simulink model "blending_tank_auto"  (R2020b)
settings: Solver=FixedStepAuto  StartTime=0.0  StopTime=Inf  RelTol=1e-3
PostLoadFcn:
  | slplc.api.loadDataTypes;
InitFcn:
  | T1_InitialValue = FB_TON.InitialValue;
  | T1_InitialValue.PRE = 20000;
  | 
  | C1_InitialValue = FB_CTU.InitialValue;
  | C1_InitialValue.PRE = 3;
StopFcn:
  | clear T1_InitialValue C1_InitialValue;
undefined symbols (not defined in the file): BOOL, DINT, OTL, REAL, slplc
libraries: simulink x3, sldrtlib x1
(part 11 of 15)

== system blending_tank_auto/PLC Controller/__Logic/Task/Program/__Logic/OTU7/Instruction_Enable/Rung-condition-in is true ==
  Enable : EnablePort
  Constant : Constant  Value=0  OutDataTypeStr=BOOL
  __CoreVarWrite : Subsystem  Tag=CoreVarWriteBlock  DisableCoverage=on  TreatAsAtomicUnit=on  mask{PLCBlockType=CoreVarWrite}
      mask init:
      | slplc.callbacks.initCoreVariable(gcb, 'write');
      mask Help: web([docroot '/plccoder/ref/__corevarwrite' '.html']);
      mask DialogControl PLCBlockTitle Prompt: Core Variable Write
  wires:
  Constant/1 -> __CoreVarWrite/1(u)

== system blending_tank_auto/PLC Controller/__Logic/Task/Program/__Logic/OTU7/RungInOverride/ForceRungInFalseRead ==
  __CoreLabelRead : Subsystem  Tag=CoreVarReadBlock  DisableCoverage=on  TreatAsAtomicUnit=on  mask{PLCBlockType=CoreLabelRead}
      mask init:
      | slplc.callbacks.initRoutineLabelRead(gcb);
      mask Help: web([docroot '/plccoder/ref/__corelabelread' '.html']);
      mask DialogControl PLCBlockTitle Prompt: Core Label Read
  Out1 : Outport  VectorParamsAs1DForOutWhenUnconnected=off
  wires:
  __CoreLabelRead/1(Out1) -> Out1/1

== system blending_tank_auto/PLC Controller/__Logic/Task/Program/__Logic/OTU8/BlockEnableRead/__CoreLabelRead ==
  DataRead : DataStoreRead  DataStoreName=x_PLCLabel__s4_3653__Block_Enable
  Out1 : Outport  VectorParamsAs1DForOutWhenUnconnected=off
  wires:
  DataRead/1 -> Out1/1

== system blending_tank_auto/PLC Controller/__Logic/Task/Program/__Logic/OTU8/Instruction_Enable/Rung-condition-in is true ==
  Enable : EnablePort
  Constant : Constant  Value=0  OutDataTypeStr=BOOL
  __CoreVarWrite : Subsystem  Tag=CoreVarWriteBlock  DisableCoverage=on  TreatAsAtomicUnit=on  mask{PLCBlockType=CoreVarWrite}
      mask init:
      | slplc.callbacks.initCoreVariable(gcb, 'write');
      mask Help: web([docroot '/plccoder/ref/__corevarwrite' '.html']);
      mask DialogControl PLCBlockTitle Prompt: Core Variable Write
  wires:
  Constant/1 -> __CoreVarWrite/1(u)

== system blending_tank_auto/PLC Controller/__Logic/Task/Program/__Logic/OTU8/RungInOverride/ForceRungInFalseRead ==
  __CoreLabelRead : Subsystem  Tag=CoreVarReadBlock  DisableCoverage=on  TreatAsAtomicUnit=on  mask{PLCBlockType=CoreLabelRead}
      mask init:
      | slplc.callbacks.initRoutineLabelRead(gcb);
      mask Help: web([docroot '/plccoder/ref/__corelabelread' '.html']);
      mask DialogControl PLCBlockTitle Prompt: Core Label Read
  Out1 : Outport  VectorParamsAs1DForOutWhenUnconnected=off
  wires:
  __CoreLabelRead/1(Out1) -> Out1/1

== system blending_tank_auto/PLC Controller/__Logic/Task/Program/__Logic/OTU9/BlockEnableRead/__CoreLabelRead ==
  DataRead : DataStoreRead  DataStoreName=x_PLCLabel__s4_3653__Block_Enable
  Out1 : Outport  VectorParamsAs1DForOutWhenUnconnected=off
  wires:
  DataRead/1 -> Out1/1

== system blending_tank_auto/PLC Controller/__Logic/Task/Program/__Logic/OTU9/Instruction_Enable/Rung-condition-in is true ==
  Enable : EnablePort
  Constant : Constant  Value=0  OutDataTypeStr=BOOL
  __CoreVarWrite : Subsystem  Tag=CoreVarWriteBlock  DisableCoverage=on  TreatAsAtomicUnit=on  mask{PLCBlockType=CoreVarWrite}
      mask init:
      | slplc.callbacks.initCoreVariable(gcb, 'write');
      mask Help: web([docroot '/plccoder/ref/__corevarwrite' '.html']);
      mask DialogControl PLCBlockTitle Prompt: Core Variable Write
  wires:
  Constant/1 -> __CoreVarWrite/1(u)

== system blending_tank_auto/PLC Controller/__Logic/Task/Program/__Logic/OTU9/RungInOverride/ForceRungInFalseRead ==
  __CoreLabelRead : Subsystem  Tag=CoreVarReadBlock  DisableCoverage=on  TreatAsAtomicUnit=on  mask{PLCBlockType=CoreLabelRead}
      mask init:
      | slplc.callbacks.initRoutineLabelRead(gcb);
      mask Help: web([docroot '/plccoder/ref/__corelabelread' '.html']);
      mask DialogControl PLCBlockTitle Prompt: Core Label Read
  Out1 : Outport  VectorParamsAs1DForOutWhenUnconnected=off
  wires:
  __CoreLabelRead/1(Out1) -> Out1/1

== system blending_tank_auto/PLC Controller/__Logic/Task/Program/__Logic/RES/BlockEnableRead/__CoreLabelRead ==
  DataRead : DataStoreRead  DataStoreName=x_PLCLabel__s4_3653__Block_Enable
  Out1 : Outport  VectorParamsAs1DForOutWhenUnconnected=off
  wires:
  DataRead/1 -> Out1/1

== system blending_tank_auto/PLC Controller/__Logic/Task/Program/__Logic/RES/Instruction_Enable/Rung-condition-in is true ==
  Enable : EnablePort
  __CoreVarRead : Subsystem  Tag=CoreVarReadBlock  DisableCoverage=on  TreatAsAtomicUnit=on  mask{PLCBlockType=CoreVarRead}
      mask init:
      | slplc.callbacks.initCoreVariable(gcb, 'read');
      mask Help: web([docroot '/plccoder/ref/__corevarread' '.html']);
      mask DialogControl PLCBlockTitle Prompt: Core Variable Read
  __CoreVarWrite : Subsystem  Tag=CoreVarWriteBlock  DisableCoverage=on  TreatAsAtomicUnit=on  mask{PLCBlockType=CoreVarWrite}
      mask init:
      | slplc.callbacks.initCoreVariable(gcb, 'write');
      mask Help: web([docroot '/plccoder/ref/__corevarwrite' '.html']);
      mask DialogControl PLCBlockTitle Prompt: Core Variable Write
  reset_function : MATLAB Function  DisableCoverage=on  TreatAsAtomicUnit=on
  wires:
  __CoreVarRead/1(y) -> reset_function/1("y ")
  reset_function/1(y) -> __CoreVarWrite/1(u)

== system blending_tank_auto/PLC Controller/__Logic/Task/Program/__Logic/RES/RungInOverride/ForceRungInFalseRead ==
  __CoreLabelRead : Subsystem  Tag=CoreVarReadBlock  DisableCoverage=on  TreatAsAtomicUnit=on  mask{PLCBlockType=CoreLabelRead}
      mask init:
      | slplc.callbacks.initRoutineLabelRead(gcb);
      mask Help: web([docroot '/plccoder/ref/__corelabelread' '.html']);
      mask DialogControl PLCBlockTitle Prompt: Core Label Read
  Out1 : Outport  VectorParamsAs1DForOutWhenUnconnected=off
  wires:
  __CoreLabelRead/1(Out1) -> Out1/1

== system blending_tank_auto/PLC Controller/__Logic/Task/Program/__Logic/RES1/BlockEnableRead/__CoreLabelRead ==
  DataRead : DataStoreRead  DataStoreName=x_PLCLabel__s4_3653__Block_Enable
  Out1 : Outport  VectorParamsAs1DForOutWhenUnconnected=off
  wires:
  DataRead/1 -> Out1/1

== system blending_tank_auto/PLC Controller/__Logic/Task/Program/__Logic/RES1/Instruction_Enable/Rung-condition-in is true ==
  Enable : EnablePort
  __CoreVarRead : Subsystem  Tag=CoreVarReadBlock  DisableCoverage=on  TreatAsAtomicUnit=on  mask{PLCBlockType=CoreVarRead}
      mask init:
      | slplc.callbacks.initCoreVariable(gcb, 'read');
      mask Help: web([docroot '/plccoder/ref/__corevarread' '.html']);
      mask DialogControl PLCBlockTitle Prompt: Core Variable Read
  __CoreVarWrite : Subsystem  Tag=CoreVarWriteBlock  DisableCoverage=on  TreatAsAtomicUnit=on  mask{PLCBlockType=CoreVarWrite}
      mask init:
      | slplc.callbacks.initCoreVariable(gcb, 'write');
      mask Help: web([docroot '/plccoder/ref/__corevarwrite' '.html']);
      mask DialogControl PLCBlockTitle Prompt: Core Variable Write
  reset_function : MATLAB Function  DisableCoverage=on  TreatAsAtomicUnit=on
  wires:
  __CoreVarRead/1(y) -> reset_function/1("y ")
  reset_function/1(y) -> __CoreVarWrite/1(u)

== system blending_tank_auto/PLC Controller/__Logic/Task/Program/__Logic/RES1/RungInOverride/ForceRungInFalseRead ==
  __CoreLabelRead : Subsystem  Tag=CoreVarReadBlock  DisableCoverage=on  TreatAsAtomicUnit=on  mask{PLCBlockType=CoreLabelRead}
      mask init:
      | slplc.callbacks.initRoutineLabelRead(gcb);
      mask Help: web([docroot '/plccoder/ref/__corelabelread' '.html']);
      mask DialogControl PLCBlockTitle Prompt: Core Label Read
  Out1 : Outport  VectorParamsAs1DForOutWhenUnconnected=off
  wires:
  __CoreLabelRead/1(Out1) -> Out1/1

== system blending_tank_auto/PLC Controller/__Logic/Task/Program/__Logic/TON/BlockEnableRead/__CoreLabelRead ==
  DataRead : DataStoreRead  DataStoreName=x_PLCLabel__s4_3653__Block_Enable
  Out1 : Outport  VectorParamsAs1DForOutWhenUnconnected=off
  wires:
  DataRead/1 -> Out1/1

== system blending_tank_auto/PLC Controller/__Logic/Task/Program/__Logic/TON/Instruction_Enable/Initialize Function ==
  Constant : Constant  Value=0  OutDataTypeStr=BOOL
  Constant1 : Constant  Value=0  OutDataTypeStr=DINT
  Event Listener : EventListener  DisableCoverage=on  EventName=reset
  VarWrite : Subsystem  DisableCoverage=on  TreatAsAtomicUnit=on  mask{PLCOperandTag=ACC, PLCOperandExpression=xxx_PLC_VAR_T1.ACC, PLCBlockType=VarWrite, PLCPOUType=VarWrite}
      mask prompts: PLCOperandTag "Operand Tag:"
      mask init:
      | slplc.callbacks.initInstruction(gcb);
      mask Help: web([docroot '/plccoder/ref/varwrite' '.html']);
      mask DialogControl PLCBlockTitle Prompt: Variable Write
      mask Display: disp(get_param(gcb, 'PLCOperandTag'));
  VarWrite1 : Subsystem  DisableCoverage=on  TreatAsAtomicUnit=on  mask{PLCOperandTag=EN, PLCOperandExpression=xxx_PLC_VAR_T1.EN, PLCBlockType=VarWrite, PLCPOUType=VarWrite}
      mask prompts: PLCOperandTag "Operand Tag:"
      mask init:
      | slplc.callbacks.initInstruction(gcb);
      mask Help: web([docroot '/plccoder/ref/varwrite' '.html']);
      mask DialogControl PLCBlockTitle Prompt: Variable Write
      mask Display: disp(get_param(gcb, 'PLCOperandTag'));
  VarWrite2 : Subsystem  DisableCoverage=on  TreatAsAtomicUnit=on  mask{PLCOperandTag=TT, PLCOperandExpression=xxx_PLC_VAR_T1.TT, PLCBlockType=VarWrite, PLCPOUType=VarWrite}
      mask prompts: PLCOperandTag "Operand Tag:"
      mask init:
      | slplc.callbacks.initInstruction(gcb);
      mask Help: web([docroot '/plccoder/ref/varwrite' '.html']);
      mask DialogControl PLCBlockTitle Prompt: Variable Write
      mask Display: disp(get_param(gcb, 'PLCOperandTag'));
  VarWrite3 : Subsystem  DisableCoverage=on  TreatAsAtomicUnit=on  mask{PLCOperandTag=DN, PLCOperandExpression=xxx_PLC_VAR_T1.DN, PLCBlockType=VarWrite, PLCPOUType=VarWrite}
      mask prompts: PLCOperandTag "Operand Tag:"
      mask init:
      | slplc.callbacks.initInstruction(gcb);
      mask Help: web([docroot '/plccoder/ref/varwrite' '.html']);
      mask DialogControl PLCBlockTitle Prompt: Variable Write
      mask Display: disp(get_param(gcb, 'PLCOperandTag'));
  wires:
  Constant/1 -> VarWrite1/1(In1), VarWrite2/1(In1), VarWrite3/1(In1)
  Constant1/1 -> VarWrite/1(In1)

== system blending_tank_auto/PLC Controller/__Logic/Task/Program/__Logic/TON/Instruction_Enable/__CoreVarRead ==
  DataRead : DataStoreRead  DataStoreName=xxx_PLC_VAR_T1
  y : Outport  VectorParamsAs1DForOutWhenUnconnected=off
  wires:
  DataRead/1 -> y/1

== system blending_tank_auto/PLC Controller/__Logic/Task/Program/__Logic/TON/Instruction_Enable/__CoreVarWrite ==
  u : Inport
  DataWrite : DataStoreWrite  DataStoreName=xxx_PLC_VAR_T1
  wires:
  u/1 -> DataWrite/1

== system blending_tank_auto/PLC Controller/__Logic/Task/Program/__Logic/TON/RungInOverride/ForceRungInFalseRead ==
  __CoreLabelRead : Subsystem  Tag=CoreVarReadBlock  DisableCoverage=on  TreatAsAtomicUnit=on  mask{PLCBlockType=CoreLabelRead}
      mask init:
      | slplc.callbacks.initRoutineLabelRead(gcb);
      mask Help: web([docroot '/plccoder/ref/__corelabelread' '.html']);
      mask DialogControl PLCBlockTitle Prompt: Core Label Read
  Out1 : Outport  VectorParamsAs1DForOutWhenUnconnected=off
  wires:
  __CoreLabelRead/1(Out1) -> Out1/1

== system blending_tank_auto/PLC Controller/__Logic/Task/Program/__Logic/XIC/BlockEnableRead/__CoreLabelRead ==
  DataRead : DataStoreRead  DataStoreName=x_PLCLabel__s4_3653__Block_Enable
  Out1 : Outport  VectorParamsAs1DForOutWhenUnconnected=off
  wires:
  DataRead/1 -> Out1/1

== system blending_tank_auto/PLC Controller/__Logic/Task/Program/__Logic/XIC/Instruction_Enable/__CoreVarRead ==
  DataRead : DataStoreRead  DataStoreName=xxx_PLC_VAR_Initialise
  y : Outport  VectorParamsAs1DForOutWhenUnconnected=off
  wires:
  DataRead/1 -> y/1

== system blending_tank_auto/PLC Controller/__Logic/Task/Program/__Logic/XIC/RungInOverride/ForceRungInFalseRead ==
  __CoreLabelRead : Subsystem  Tag=CoreVarReadBlock  DisableCoverage=on  TreatAsAtomicUnit=on  mask{PLCBlockType=CoreLabelRead}
      mask init:
      | slplc.callbacks.initRoutineLabelRead(gcb);
      mask Help: web([docroot '/plccoder/ref/__corelabelread' '.html']);
      mask DialogControl PLCBlockTitle Prompt: Core Label Read
  Out1 : Outport  VectorParamsAs1DForOutWhenUnconnected=off
  wires:
  __CoreLabelRead/1(Out1) -> Out1/1

== system blending_tank_auto/PLC Controller/__Logic/Task/Program/__Logic/XIC1/BlockEnableRead/__CoreLabelRead ==
  DataRead : DataStoreRead  DataStoreName=x_PLCLabel__s4_3653__Block_Enable
  Out1 : Outport  VectorParamsAs1DForOutWhenUnconnected=off
  wires:
  DataRead/1 -> Out1/1

== system blending_tank_auto/PLC Controller/__Logic/Task/Program/__Logic/XIC1/Instruction_Enable/__CoreVarRead ==
  DataRead : DataStoreRead  DataStoreName=xxx_PLC_VAR_M0
  y : Outport  VectorParamsAs1DForOutWhenUnconnected=off
  wires:
  DataRead/1 -> y/1

== system blending_tank_auto/PLC Controller/__Logic/Task/Program/__Logic/XIC1/RungInOverride/ForceRungInFalseRead ==
  __CoreLabelRead : Subsystem  Tag=CoreVarReadBlock  DisableCoverage=on  TreatAsAtomicUnit=on  mask{PLCBlockType=CoreLabelRead}
      mask init:
      | slplc.callbacks.initRoutineLabelRead(gcb);
      mask Help: web([docroot '/plccoder/ref/__corelabelread' '.html']);
      mask DialogControl PLCBlockTitle Prompt: Core Label Read
  Out1 : Outport  VectorParamsAs1DForOutWhenUnconnected=off
  wires:
  __CoreLabelRead/1(Out1) -> Out1/1

== system blending_tank_auto/PLC Controller/__Logic/Task/Program/__Logic/XIC10/BlockEnableRead/__CoreLabelRead ==
  DataRead : DataStoreRead  DataStoreName=x_PLCLabel__s4_3653__Block_Enable
  Out1 : Outport  VectorParamsAs1DForOutWhenUnconnected=off
  wires:
  DataRead/1 -> Out1/1

== system blending_tank_auto/PLC Controller/__Logic/Task/Program/__Logic/XIC10/Instruction_Enable/__CoreVarRead ==
  DataRead : DataStoreRead  DataStoreName=xxx_PLC_VAR_M6
  y : Outport  VectorParamsAs1DForOutWhenUnconnected=off
  wires:
  DataRead/1 -> y/1

== system blending_tank_auto/PLC Controller/__Logic/Task/Program/__Logic/XIC10/RungInOverride/ForceRungInFalseRead ==
  __CoreLabelRead : Subsystem  Tag=CoreVarReadBlock  DisableCoverage=on  TreatAsAtomicUnit=on  mask{PLCBlockType=CoreLabelRead}
      mask init:
      | slplc.callbacks.initRoutineLabelRead(gcb);
      mask Help: web([docroot '/plccoder/ref/__corelabelread' '.html']);
      mask DialogControl PLCBlockTitle Prompt: Core Label Read
  Out1 : Outport  VectorParamsAs1DForOutWhenUnconnected=off
  wires:
  __CoreLabelRead/1(Out1) -> Out1/1

== system blending_tank_auto/PLC Controller/__Logic/Task/Program/__Logic/XIC11/BlockEnableRead/__CoreLabelRead ==
  DataRead : DataStoreRead  DataStoreName=x_PLCLabel__s4_3653__Block_Enable
  Out1 : Outport  VectorParamsAs1DForOutWhenUnconnected=off
  wires:
  DataRead/1 -> Out1/1

== system blending_tank_auto/PLC Controller/__Logic/Task/Program/__Logic/XIC11/Instruction_Enable/__CoreVarRead ==
  DataRead : DataStoreRead  DataStoreName=xxx_PLC_VAR_M7
  y : Outport  VectorParamsAs1DForOutWhenUnconnected=off
  wires:
  DataRead/1 -> y/1

== system blending_tank_auto/PLC Controller/__Logic/Task/Program/__Logic/XIC11/RungInOverride/ForceRungInFalseRead ==
  __CoreLabelRead : Subsystem  Tag=CoreVarReadBlock  DisableCoverage=on  TreatAsAtomicUnit=on  mask{PLCBlockType=CoreLabelRead}
      mask init:
      | slplc.callbacks.initRoutineLabelRead(gcb);
      mask Help: web([docroot '/plccoder/ref/__corelabelread' '.html']);
      mask DialogControl PLCBlockTitle Prompt: Core Label Read
  Out1 : Outport  VectorParamsAs1DForOutWhenUnconnected=off
  wires:
  __CoreLabelRead/1(Out1) -> Out1/1

== system blending_tank_auto/PLC Controller/__Logic/Task/Program/__Logic/XIC12/BlockEnableRead/__CoreLabelRead ==
  DataRead : DataStoreRead  DataStoreName=x_PLCLabel__s4_3653__Block_Enable
  Out1 : Outport  VectorParamsAs1DForOutWhenUnconnected=off
  wires:
  DataRead/1 -> Out1/1

== system blending_tank_auto/PLC Controller/__Logic/Task/Program/__Logic/XIC12/Instruction_Enable/__CoreVarRead ==
  DataRead : DataStoreRead  DataStoreName=xxx_PLC_VAR_M5
  y : Outport  VectorParamsAs1DForOutWhenUnconnected=off
  wires:
  DataRead/1 -> y/1

== system blending_tank_auto/PLC Controller/__Logic/Task/Program/__Logic/XIC12/RungInOverride/ForceRungInFalseRead ==
  __CoreLabelRead : Subsystem  Tag=CoreVarReadBlock  DisableCoverage=on  TreatAsAtomicUnit=on  mask{PLCBlockType=CoreLabelRead}
      mask init:
      | slplc.callbacks.initRoutineLabelRead(gcb);
      mask Help: web([docroot '/plccoder/ref/__corelabelread' '.html']);
      mask DialogControl PLCBlockTitle Prompt: Core Label Read
  Out1 : Outport  VectorParamsAs1DForOutWhenUnconnected=off
  wires:
  __CoreLabelRead/1(Out1) -> Out1/1

== system blending_tank_auto/PLC Controller/__Logic/Task/Program/__Logic/XIC13/BlockEnableRead/__CoreLabelRead ==
  DataRead : DataStoreRead  DataStoreName=x_PLCLabel__s4_3653__Block_Enable
  Out1 : Outport  VectorParamsAs1DForOutWhenUnconnected=off
  wires:
  DataRead/1 -> Out1/1

== system blending_tank_auto/PLC Controller/__Logic/Task/Program/__Logic/XIC13/Instruction_Enable/__CoreVarRead ==
  DataRead : DataStoreRead  DataStoreName=xxx_PLC_VAR_M2
  y : Outport  VectorParamsAs1DForOutWhenUnconnected=off
  wires:
  DataRead/1 -> y/1

== system blending_tank_auto/PLC Controller/__Logic/Task/Program/__Logic/XIC13/RungInOverride/ForceRungInFalseRead ==
  __CoreLabelRead : Subsystem  Tag=CoreVarReadBlock  DisableCoverage=on  TreatAsAtomicUnit=on  mask{PLCBlockType=CoreLabelRead}
      mask init:
      | slplc.callbacks.initRoutineLabelRead(gcb);
      mask Help: web([docroot '/plccoder/ref/__corelabelread' '.html']);
      mask DialogControl PLCBlockTitle Prompt: Core Label Read
  Out1 : Outport  VectorParamsAs1DForOutWhenUnconnected=off
  wires:
  __CoreLabelRead/1(Out1) -> Out1/1

== system blending_tank_auto/PLC Controller/__Logic/Task/Program/__Logic/XIC14/BlockEnableRead/__CoreLabelRead ==
  DataRead : DataStoreRead  DataStoreName=x_PLCLabel__s4_3653__Block_Enable
  Out1 : Outport  VectorParamsAs1DForOutWhenUnconnected=off
  wires:
  DataRead/1 -> Out1/1

== system blending_tank_auto/PLC Controller/__Logic/Task/Program/__Logic/XIC14/Instruction_Enable/__CoreVarRead ==
  DataRead : DataStoreRead  DataStoreName=xxx_PLC_VAR_M3
  y : Outport  VectorParamsAs1DForOutWhenUnconnected=off
  wires:
  DataRead/1 -> y/1

== system blending_tank_auto/PLC Controller/__Logic/Task/Program/__Logic/XIC14/RungInOverride/ForceRungInFalseRead ==
  __CoreLabelRead : Subsystem  Tag=CoreVarReadBlock  DisableCoverage=on  TreatAsAtomicUnit=on  mask{PLCBlockType=CoreLabelRead}
      mask init:
      | slplc.callbacks.initRoutineLabelRead(gcb);
      mask Help: web([docroot '/plccoder/ref/__corelabelread' '.html']);
      mask DialogControl PLCBlockTitle Prompt: Core Label Read
  Out1 : Outport  VectorParamsAs1DForOutWhenUnconnected=off
  wires:
  __CoreLabelRead/1(Out1) -> Out1/1

== system blending_tank_auto/PLC Controller/__Logic/Task/Program/__Logic/XIC15/BlockEnableRead/__CoreLabelRead ==
  DataRead : DataStoreRead  DataStoreName=x_PLCLabel__s4_3653__Block_Enable
  Out1 : Outport  VectorParamsAs1DForOutWhenUnconnected=off
  wires:
  DataRead/1 -> Out1/1

== system blending_tank_auto/PLC Controller/__Logic/Task/Program/__Logic/XIC15/Instruction_Enable/__CoreVarRead ==
  DataRead : DataStoreRead  DataStoreName=xxx_PLC_VAR_M4
  y : Outport  VectorParamsAs1DForOutWhenUnconnected=off
  wires:
  DataRead/1 -> y/1

== system blending_tank_auto/PLC Controller/__Logic/Task/Program/__Logic/XIC15/RungInOverride/ForceRungInFalseRead ==
  __CoreLabelRead : Subsystem  Tag=CoreVarReadBlock  DisableCoverage=on  TreatAsAtomicUnit=on  mask{PLCBlockType=CoreLabelRead}
      mask init:
      | slplc.callbacks.initRoutineLabelRead(gcb);
      mask Help: web([docroot '/plccoder/ref/__corelabelread' '.html']);
      mask DialogControl PLCBlockTitle Prompt: Core Label Read
  Out1 : Outport  VectorParamsAs1DForOutWhenUnconnected=off
  wires:
  __CoreLabelRead/1(Out1) -> Out1/1

== system blending_tank_auto/PLC Controller/__Logic/Task/Program/__Logic/XIC16/BlockEnableRead/__CoreLabelRead ==
  DataRead : DataStoreRead  DataStoreName=x_PLCLabel__s4_3653__Block_Enable
  Out1 : Outport  VectorParamsAs1DForOutWhenUnconnected=off
  wires:
  DataRead/1 -> Out1/1

== system blending_tank_auto/PLC Controller/__Logic/Task/Program/__Logic/XIC16/Instruction_Enable/__CoreVarRead ==
  DataRead : DataStoreRead  DataStoreName=xxx_PLC_VAR_M1
  y : Outport  VectorParamsAs1DForOutWhenUnconnected=off
  wires:
  DataRead/1 -> y/1

== system blending_tank_auto/PLC Controller/__Logic/Task/Program/__Logic/XIC16/RungInOverride/ForceRungInFalseRead ==
  __CoreLabelRead : Subsystem  Tag=CoreVarReadBlock  DisableCoverage=on  TreatAsAtomicUnit=on  mask{PLCBlockType=CoreLabelRead}
      mask init:
      | slplc.callbacks.initRoutineLabelRead(gcb);
      mask Help: web([docroot '/plccoder/ref/__corelabelread' '.html']);
      mask DialogControl PLCBlockTitle Prompt: Core Label Read
  Out1 : Outport  VectorParamsAs1DForOutWhenUnconnected=off
  wires:
  __CoreLabelRead/1(Out1) -> Out1/1

== system blending_tank_auto/PLC Controller/__Logic/Task/Program/__Logic/XIC17/BlockEnableRead/__CoreLabelRead ==
  DataRead : DataStoreRead  DataStoreName=x_PLCLabel__s4_3653__Block_Enable
  Out1 : Outport  VectorParamsAs1DForOutWhenUnconnected=off
  wires:
  DataRead/1 -> Out1/1

== system blending_tank_auto/PLC Controller/__Logic/Task/Program/__Logic/XIC17/Instruction_Enable/__CoreVarRead ==
  DataRead : DataStoreRead  DataStoreName=xxx_PLC_VAR_M6
  y : Outport  VectorParamsAs1DForOutWhenUnconnected=off
  wires:
  DataRead/1 -> y/1

== system blending_tank_auto/PLC Controller/__Logic/Task/Program/__Logic/XIC17/RungInOverride/ForceRungInFalseRead ==
  __CoreLabelRead : Subsystem  Tag=CoreVarReadBlock  DisableCoverage=on  TreatAsAtomicUnit=on  mask{PLCBlockType=CoreLabelRead}
      mask init:
      | slplc.callbacks.initRoutineLabelRead(gcb);
      mask Help: web([docroot '/plccoder/ref/__corelabelread' '.html']);
      mask DialogControl PLCBlockTitle Prompt: Core Label Read
  Out1 : Outport  VectorParamsAs1DForOutWhenUnconnected=off
  wires:
  __CoreLabelRead/1(Out1) -> Out1/1

== system blending_tank_auto/PLC Controller/__Logic/Task/Program/__Logic/XIC18/BlockEnableRead/__CoreLabelRead ==
  DataRead : DataStoreRead  DataStoreName=x_PLCLabel__s4_3653__Block_Enable
  Out1 : Outport  VectorParamsAs1DForOutWhenUnconnected=off
  wires:
  DataRead/1 -> Out1/1

== system blending_tank_auto/PLC Controller/__Logic/Task/Program/__Logic/XIC18/Instruction_Enable/__CoreVarRead ==
  DataRead : DataStoreRead  DataStoreName=xxx_PLC_VAR_M5
  y : Outport  VectorParamsAs1DForOutWhenUnconnected=off
  wires:
  DataRead/1 -> y/1

== system blending_tank_auto/PLC Controller/__Logic/Task/Program/__Logic/XIC18/RungInOverride/ForceRungInFalseRead ==
  __CoreLabelRead : Subsystem  Tag=CoreVarReadBlock  DisableCoverage=on  TreatAsAtomicUnit=on  mask{PLCBlockType=CoreLabelRead}
      mask init:
      | slplc.callbacks.initRoutineLabelRead(gcb);
      mask Help: web([docroot '/plccoder/ref/__corelabelread' '.html']);
      mask DialogControl PLCBlockTitle Prompt: Core Label Read
  Out1 : Outport  VectorParamsAs1DForOutWhenUnconnected=off
  wires:
  __CoreLabelRead/1(Out1) -> Out1/1

== system blending_tank_auto/PLC Controller/__Logic/Task/Program/__Logic/XIC19/BlockEnableRead/__CoreLabelRead ==
  DataRead : DataStoreRead  DataStoreName=x_PLCLabel__s4_3653__Block_Enable
  Out1 : Outport  VectorParamsAs1DForOutWhenUnconnected=off
  wires:
  DataRead/1 -> Out1/1

== system blending_tank_auto/PLC Controller/__Logic/Task/Program/__Logic/XIC19/Instruction_Enable/__CoreVarRead ==
  DataRead : DataStoreRead  DataStoreName=xxx_PLC_VAR_M6
  y : Outport  VectorParamsAs1DForOutWhenUnconnected=off
  wires:
  DataRead/1 -> y/1

== system blending_tank_auto/PLC Controller/__Logic/Task/Program/__Logic/XIC19/RungInOverride/ForceRungInFalseRead ==
  __CoreLabelRead : Subsystem  Tag=CoreVarReadBlock  DisableCoverage=on  TreatAsAtomicUnit=on  mask{PLCBlockType=CoreLabelRead}
      mask init:
      | slplc.callbacks.initRoutineLabelRead(gcb);
      mask Help: web([docroot '/plccoder/ref/__corelabelread' '.html']);
      mask DialogControl PLCBlockTitle Prompt: Core Label Read
  Out1 : Outport  VectorParamsAs1DForOutWhenUnconnected=off
  wires:
  __CoreLabelRead/1(Out1) -> Out1/1

== system blending_tank_auto/PLC Controller/__Logic/Task/Program/__Logic/XIC2/BlockEnableRead/__CoreLabelRead ==
  DataRead : DataStoreRead  DataStoreName=x_PLCLabel__s4_3653__Block_Enable
  Out1 : Outport  VectorParamsAs1DForOutWhenUnconnected=off
  wires:
  DataRead/1 -> Out1/1

== system blending_tank_auto/PLC Controller/__Logic/Task/Program/__Logic/XIC2/Instruction_Enable/__CoreVarRead ==
  DataRead : DataStoreRead  DataStoreName=xxx_PLC_VAR_Start_Button
  y : Outport  VectorParamsAs1DForOutWhenUnconnected=off
  wires:
  DataRead/1 -> y/1

== system blending_tank_auto/PLC Controller/__Logic/Task/Program/__Logic/XIC2/RungInOverride/ForceRungInFalseRead ==
  __CoreLabelRead : Subsystem  Tag=CoreVarReadBlock  DisableCoverage=on  TreatAsAtomicUnit=on  mask{PLCBlockType=CoreLabelRead}
      mask init:
      | slplc.callbacks.initRoutineLabelRead(gcb);
      mask Help: web([docroot '/plccoder/ref/__corelabelread' '.html']);
      mask DialogControl PLCBlockTitle Prompt: Core Label Read
  Out1 : Outport  VectorParamsAs1DForOutWhenUnconnected=off
  wires:
  __CoreLabelRead/1(Out1) -> Out1/1

== system blending_tank_auto/PLC Controller/__Logic/Task/Program/__Logic/XIC20/BlockEnableRead/__CoreLabelRead ==
  DataRead : DataStoreRead  DataStoreName=x_PLCLabel__s4_3653__Block_Enable
  Out1 : Outport  VectorParamsAs1DForOutWhenUnconnected=off
  wires:
  DataRead/1 -> Out1/1

== system blending_tank_auto/PLC Controller/__Logic/Task/Program/__Logic/XIC20/Instruction_Enable/__CoreVarRead ==
  DataRead : DataStoreRead  DataStoreName=xxx_PLC_VAR_M7
  y : Outport  VectorParamsAs1DForOutWhenUnconnected=off
  wires:
  DataRead/1 -> y/1

== system blending_tank_auto/PLC Controller/__Logic/Task/Program/__Logic/XIC20/RungInOverride/ForceRungInFalseRead ==
  __CoreLabelRead : Subsystem  Tag=CoreVarReadBlock  DisableCoverage=on  TreatAsAtomicUnit=on  mask{PLCBlockType=CoreLabelRead}
      mask init:
      | slplc.callbacks.initRoutineLabelRead(gcb);
      mask Help: web([docroot '/plccoder/ref/__corelabelread' '.html']);
      mask DialogControl PLCBlockTitle Prompt: Core Label Read
  Out1 : Outport  VectorParamsAs1DForOutWhenUnconnected=off
  wires:
  __CoreLabelRead/1(Out1) -> Out1/1

== system blending_tank_auto/PLC Controller/__Logic/Task/Program/__Logic/XIC21/BlockEnableRead/__CoreLabelRead ==
  DataRead : DataStoreRead  DataStoreName=x_PLCLabel__s4_3653__Block_Enable
  Out1 : Outport  VectorParamsAs1DForOutWhenUnconnected=off
  wires:
  DataRead/1 -> Out1/1

== system blending_tank_auto/PLC Controller/__Logic/Task/Program/__Logic/XIC21/Instruction_Enable/__CoreVarRead ==
  DataRead : DataStoreRead  DataStoreName=xxx_PLC_VAR_C1  DataStoreElements=xxx_PLC_VAR_C1.DN
  y : Outport  VectorParamsAs1DForOutWhenUnconnected=off
  wires:
  DataRead/1 -> y/1

== system blending_tank_auto/PLC Controller/__Logic/Task/Program/__Logic/XIC21/RungInOverride/ForceRungInFalseRead ==
  __CoreLabelRead : Subsystem  Tag=CoreVarReadBlock  DisableCoverage=on  TreatAsAtomicUnit=on  mask{PLCBlockType=CoreLabelRead}
      mask init:
      | slplc.callbacks.initRoutineLabelRead(gcb);
      mask Help: web([docroot '/plccoder/ref/__corelabelread' '.html']);
      mask DialogControl PLCBlockTitle Prompt: Core Label Read
  Out1 : Outport  VectorParamsAs1DForOutWhenUnconnected=off
  wires:
  __CoreLabelRead/1(Out1) -> Out1/1

== system blending_tank_auto/PLC Controller/__Logic/Task/Program/__Logic/XIC22/BlockEnableRead/__CoreLabelRead ==
  DataRead : DataStoreRead  DataStoreName=x_PLCLabel__s4_3653__Block_Enable
  Out1 : Outport  VectorParamsAs1DForOutWhenUnconnected=off
  wires:
  DataRead/1 -> Out1/1

== system blending_tank_auto/PLC Controller/__Logic/Task/Program/__Logic/XIC22/Instruction_Enable/__CoreVarRead ==
  DataRead : DataStoreRead  DataStoreName=xxx_PLC_VAR_M0
  y : Outport  VectorParamsAs1DForOutWhenUnconnected=off
  wires:
  DataRead/1 -> y/1

== system blending_tank_auto/PLC Controller/__Logic/Task/Program/__Logic/XIC22/RungInOverride/ForceRungInFalseRead ==
  __CoreLabelRead : Subsystem  Tag=CoreVarReadBlock  DisableCoverage=on  TreatAsAtomicUnit=on  mask{PLCBlockType=CoreLabelRead}
      mask init:
      | slplc.callbacks.initRoutineLabelRead(gcb);
      mask Help: web([docroot '/plccoder/ref/__corelabelread' '.html']);
      mask DialogControl PLCBlockTitle Prompt: Core Label Read
  Out1 : Outport  VectorParamsAs1DForOutWhenUnconnected=off
  wires:
  __CoreLabelRead/1(Out1) -> Out1/1

== system blending_tank_auto/PLC Controller/__Logic/Task/Program/__Logic/XIC23/BlockEnableRead/__CoreLabelRead ==
  DataRead : DataStoreRead  DataStoreName=x_PLCLabel__s4_3653__Block_Enable
  Out1 : Outport  VectorParamsAs1DForOutWhenUnconnected=off
  wires:
  DataRead/1 -> Out1/1

== system blending_tank_auto/PLC Controller/__Logic/Task/Program/__Logic/XIC23/Instruction_Enable/__CoreVarRead ==
  DataRead : DataStoreRead  DataStoreName=xxx_PLC_VAR_M1
  y : Outport  VectorParamsAs1DForOutWhenUnconnected=off
  wires:
  DataRead/1 -> y/1

== system blending_tank_auto/PLC Controller/__Logic/Task/Program/__Logic/XIC23/RungInOverride/ForceRungInFalseRead ==
  __CoreLabelRead : Subsystem  Tag=CoreVarReadBlock  DisableCoverage=on  TreatAsAtomicUnit=on  mask{PLCBlockType=CoreLabelRead}
      mask init:
      | slplc.callbacks.initRoutineLabelRead(gcb);
      mask Help: web([docroot '/plccoder/ref/__corelabelread' '.html']);
      mask DialogControl PLCBlockTitle Prompt: Core Label Read
  Out1 : Outport  VectorParamsAs1DForOutWhenUnconnected=off
  wires:
  __CoreLabelRead/1(Out1) -> Out1/1

== system blending_tank_auto/PLC Controller/__Logic/Task/Program/__Logic/XIC3/BlockEnableRead/__CoreLabelRead ==
  DataRead : DataStoreRead  DataStoreName=x_PLCLabel__s4_3653__Block_Enable
  Out1 : Outport  VectorParamsAs1DForOutWhenUnconnected=off
  wires:
  DataRead/1 -> Out1/1

== system blending_tank_auto/PLC Controller/__Logic/Task/Program/__Logic/XIC3/Instruction_Enable/__CoreVarRead ==
  DataRead : DataStoreRead  DataStoreName=xxx_PLC_VAR_M1
  y : Outport  VectorParamsAs1DForOutWhenUnconnected=off
  wires:
  DataRead/1 -> y/1

== system blending_tank_auto/PLC Controller/__Logic/Task/Program/__Logic/XIC3/RungInOverride/ForceRungInFalseRead ==
  __CoreLabelRead : Subsystem  Tag=CoreVarReadBlock  DisableCoverage=on  TreatAsAtomicUnit=on  mask{PLCBlockType=CoreLabelRead}
      mask init:
      | slplc.callbacks.initRoutineLabelRead(gcb);
      mask Help: web([docroot '/plccoder/ref/__corelabelread' '.html']);
      mask DialogControl PLCBlockTitle Prompt: Core Label Read
  Out1 : Outport  VectorParamsAs1DForOutWhenUnconnected=off
  wires:
  __CoreLabelRead/1(Out1) -> Out1/1

== system blending_tank_auto/PLC Controller/__Logic/Task/Program/__Logic/XIC4/BlockEnableRead/__CoreLabelRead ==
  DataRead : DataStoreRead  DataStoreName=x_PLCLabel__s4_3653__Block_Enable
  Out1 : Outport  VectorParamsAs1DForOutWhenUnconnected=off
  wires:
  DataRead/1 -> Out1/1

== system blending_tank_auto/PLC Controller/__Logic/Task/Program/__Logic/XIC4/Instruction_Enable/__CoreVarRead ==
  DataRead : DataStoreRead  DataStoreName=xxx_PLC_VAR_M2
  y : Outport  VectorParamsAs1DForOutWhenUnconnected=off
  wires:
  DataRead/1 -> y/1

== system blending_tank_auto/PLC Controller/__Logic/Task/Program/__Logic/XIC4/RungInOverride/ForceRungInFalseRead ==
  __CoreLabelRead : Subsystem  Tag=CoreVarReadBlock  DisableCoverage=on  TreatAsAtomicUnit=on  mask{PLCBlockType=CoreLabelRead}
      mask init:
      | slplc.callbacks.initRoutineLabelRead(gcb);
      mask Help: web([docroot '/plccoder/ref/__corelabelread' '.html']);
      mask DialogControl PLCBlockTitle Prompt: Core Label Read
  Out1 : Outport  VectorParamsAs1DForOutWhenUnconnected=off
  wires:
  __CoreLabelRead/1(Out1) -> Out1/1

== system blending_tank_auto/PLC Controller/__Logic/Task/Program/__Logic/XIC5/BlockEnableRead/__CoreLabelRead ==
  DataRead : DataStoreRead  DataStoreName=x_PLCLabel__s4_3653__Block_Enable
  Out1 : Outport  VectorParamsAs1DForOutWhenUnconnected=off
  wires:
  DataRead/1 -> Out1/1

== system blending_tank_auto/PLC Controller/__Logic/Task/Program/__Logic/XIC5/Instruction_Enable/__CoreVarRead ==
  DataRead : DataStoreRead  DataStoreName=xxx_PLC_VAR_M3
  y : Outport  VectorParamsAs1DForOutWhenUnconnected=off
  wires:
  DataRead/1 -> y/1

== system blending_tank_auto/PLC Controller/__Logic/Task/Program/__Logic/XIC5/RungInOverride/ForceRungInFalseRead ==
  __CoreLabelRead : Subsystem  Tag=CoreVarReadBlock  DisableCoverage=on  TreatAsAtomicUnit=on  mask{PLCBlockType=CoreLabelRead}
      mask init:
      | slplc.callbacks.initRoutineLabelRead(gcb);
      mask Help: web([docroot '/plccoder/ref/__corelabelread' '.html']);
      mask DialogControl PLCBlockTitle Prompt: Core Label Read
  Out1 : Outport  VectorParamsAs1DForOutWhenUnconnected=off
  wires:
  __CoreLabelRead/1(Out1) -> Out1/1

== system blending_tank_auto/PLC Controller/__Logic/Task/Program/__Logic/XIC6/BlockEnableRead/__CoreLabelRead ==
  DataRead : DataStoreRead  DataStoreName=x_PLCLabel__s4_3653__Block_Enable
  Out1 : Outport  VectorParamsAs1DForOutWhenUnconnected=off
  wires:
  DataRead/1 -> Out1/1

== system blending_tank_auto/PLC Controller/__Logic/Task/Program/__Logic/XIC6/Instruction_Enable/__CoreVarRead ==
  DataRead : DataStoreRead  DataStoreName=xxx_PLC_VAR_M4
  y : Outport  VectorParamsAs1DForOutWhenUnconnected=off
  wires:
  DataRead/1 -> y/1

== system blending_tank_auto/PLC Controller/__Logic/Task/Program/__Logic/XIC6/RungInOverride/ForceRungInFalseRead ==
  __CoreLabelRead : Subsystem  Tag=CoreVarReadBlock  DisableCoverage=on  TreatAsAtomicUnit=on  mask{PLCBlockType=CoreLabelRead}
      mask init:
      | slplc.callbacks.initRoutineLabelRead(gcb);
      mask Help: web([docroot '/plccoder/ref/__corelabelread' '.html']);
      mask DialogControl PLCBlockTitle Prompt: Core Label Read
  Out1 : Outport  VectorParamsAs1DForOutWhenUnconnected=off
  wires:
  __CoreLabelRead/1(Out1) -> Out1/1

== system blending_tank_auto/PLC Controller/__Logic/Task/Program/__Logic/XIC7/BlockEnableRead/__CoreLabelRead ==
  DataRead : DataStoreRead  DataStoreName=x_PLCLabel__s4_3653__Block_Enable
  Out1 : Outport  VectorParamsAs1DForOutWhenUnconnected=off
  wires:
  DataRead/1 -> Out1/1

== system blending_tank_auto/PLC Controller/__Logic/Task/Program/__Logic/XIC7/Instruction_Enable/__CoreVarRead ==
  DataRead : DataStoreRead  DataStoreName=xxx_PLC_VAR_M5
  y : Outport  VectorParamsAs1DForOutWhenUnconnected=off
  wires:
  DataRead/1 -> y/1

== system blending_tank_auto/PLC Controller/__Logic/Task/Program/__Logic/XIC7/RungInOverride/ForceRungInFalseRead ==
  __CoreLabelRead : Subsystem  Tag=CoreVarReadBlock  DisableCoverage=on  TreatAsAtomicUnit=on  mask{PLCBlockType=CoreLabelRead}
      mask init:
      | slplc.callbacks.initRoutineLabelRead(gcb);
      mask Help: web([docroot '/plccoder/ref/__corelabelread' '.html']);
      mask DialogControl PLCBlockTitle Prompt: Core Label Read
  Out1 : Outport  VectorParamsAs1DForOutWhenUnconnected=off
  wires:
  __CoreLabelRead/1(Out1) -> Out1/1

== system blending_tank_auto/PLC Controller/__Logic/Task/Program/__Logic/XIC8/BlockEnableRead/__CoreLabelRead ==
  DataRead : DataStoreRead  DataStoreName=x_PLCLabel__s4_3653__Block_Enable
  Out1 : Outport  VectorParamsAs1DForOutWhenUnconnected=off
  wires:
  DataRead/1 -> Out1/1

== system blending_tank_auto/PLC Controller/__Logic/Task/Program/__Logic/XIC8/Instruction_Enable/__CoreVarRead ==
  DataRead : DataStoreRead  DataStoreName=xxx_PLC_VAR_T1  DataStoreElements=xxx_PLC_VAR_T1.DN
  y : Outport  VectorParamsAs1DForOutWhenUnconnected=off
  wires:
  DataRead/1 -> y/1

== system blending_tank_auto/PLC Controller/__Logic/Task/Program/__Logic/XIC8/RungInOverride/ForceRungInFalseRead ==
  __CoreLabelRead : Subsystem  Tag=CoreVarReadBlock  DisableCoverage=on  TreatAsAtomicUnit=on  mask{PLCBlockType=CoreLabelRead}
      mask init:
      | slplc.callbacks.initRoutineLabelRead(gcb);
      mask Help: web([docroot '/plccoder/ref/__corelabelread' '.html']);
      mask DialogControl PLCBlockTitle Prompt: Core Label Read
  Out1 : Outport  VectorParamsAs1DForOutWhenUnconnected=off
  wires:
  __CoreLabelRead/1(Out1) -> Out1/1

== system blending_tank_auto/PLC Controller/__Logic/Task/Program/__Logic/XIC9/BlockEnableRead/__CoreLabelRead ==
  DataRead : DataStoreRead  DataStoreName=x_PLCLabel__s4_3653__Block_Enable
  Out1 : Outport  VectorParamsAs1DForOutWhenUnconnected=off
  wires:
  DataRead/1 -> Out1/1

== system blending_tank_auto/PLC Controller/__Logic/Task/Program/__Logic/XIC9/Instruction_Enable/__CoreVarRead ==
  DataRead : DataStoreRead  DataStoreName=xxx_PLC_VAR_Initialise
  y : Outport  VectorParamsAs1DForOutWhenUnconnected=off
  wires:
  DataRead/1 -> y/1

== system blending_tank_auto/PLC Controller/__Logic/Task/Program/__Logic/XIC9/RungInOverride/ForceRungInFalseRead ==
  __CoreLabelRead : Subsystem  Tag=CoreVarReadBlock  DisableCoverage=on  TreatAsAtomicUnit=on  mask{PLCBlockType=CoreLabelRead}
      mask init:
      | slplc.callbacks.initRoutineLabelRead(gcb);
      mask Help: web([docroot '/plccoder/ref/__corelabelread' '.html']);
      mask DialogControl PLCBlockTitle Prompt: Core Label Read
  Out1 : Outport  VectorParamsAs1DForOutWhenUnconnected=off
  wires:
  __CoreLabelRead/1(Out1) -> Out1/1

== system blending_tank_auto/PLC Controller/__Logic/Task/Program/__Logic/XIO/BlockEnableRead/__CoreLabelRead ==
  DataRead : DataStoreRead  DataStoreName=x_PLCLabel__s4_3653__Block_Enable
  Out1 : Outport  VectorParamsAs1DForOutWhenUnconnected=off
  wires:
  DataRead/1 -> Out1/1

== system blending_tank_auto/PLC Controller/__Logic/Task/Program/__Logic/XIO/Instruction_Enable/__CoreVarRead ==
  DataRead : DataStoreRead  DataStoreName=xxx_PLC_VAR_Running
  y : Outport  VectorParamsAs1DForOutWhenUnconnected=off
  wires:
  DataRead/1 -> y/1

== system blending_tank_auto/PLC Controller/__Logic/Task/Program/__Logic/XIO/RungInOverride/ForceRungInFalseRead ==
  __CoreLabelRead : Subsystem  Tag=CoreVarReadBlock  DisableCoverage=on  TreatAsAtomicUnit=on  mask{PLCBlockType=CoreLabelRead}
      mask init:
      | slplc.callbacks.initRoutineLabelRead(gcb);
      mask Help: web([docroot '/plccoder/ref/__corelabelread' '.html']);
      mask DialogControl PLCBlockTitle Prompt: Core Label Read
  Out1 : Outport  VectorParamsAs1DForOutWhenUnconnected=off
  wires:
  __CoreLabelRead/1(Out1) -> Out1/1

== system blending_tank_auto/PLC Controller/__Logic/Task/Program/__Logic/XIO1/BlockEnableRead/__CoreLabelRead ==
  DataRead : DataStoreRead  DataStoreName=x_PLCLabel__s4_3653__Block_Enable
  Out1 : Outport  VectorParamsAs1DForOutWhenUnconnected=off
  wires:
  DataRead/1 -> Out1/1

== system blending_tank_auto/PLC Controller/__Logic/Task/Program/__Logic/XIO1/Instruction_Enable/__CoreVarRead ==
  DataRead : DataStoreRead  DataStoreName=xxx_PLC_VAR_C1  DataStoreElements=xxx_PLC_VAR_C1.DN
  y : Outport  VectorParamsAs1DForOutWhenUnconnected=off
  wires:
  DataRead/1 -> y/1

== system blending_tank_auto/PLC Controller/__Logic/Task/Program/__Logic/XIO1/RungInOverride/ForceRungInFalseRead ==
  __CoreLabelRead : Subsystem  Tag=CoreVarReadBlock  DisableCoverage=on  TreatAsAtomicUnit=on  mask{PLCBlockType=CoreLabelRead}
      mask init:
      | slplc.callbacks.initRoutineLabelRead(gcb);
      mask Help: web([docroot '/plccoder/ref/__corelabelread' '.html']);
      mask DialogControl PLCBlockTitle Prompt: Core Label Read
  Out1 : Outport  VectorParamsAs1DForOutWhenUnconnected=off
  wires:
  __CoreLabelRead/1(Out1) -> Out1/1

== system blending_tank_auto/PLC Controller/__Logic/Task/Program/__Logic/CTU/Instruction_Enable/Initialize Function/VarWrite1 ==
  In1 : Inport
  __CoreVarWrite : Subsystem  Tag=CoreVarWriteBlock  DisableCoverage=on  TreatAsAtomicUnit=on  mask{PLCBlockType=CoreVarWrite}
      mask init:
      | slplc.callbacks.initCoreVariable(gcb, 'write');
      mask Help: web([docroot '/plccoder/ref/__corevarwrite' '.html']);
      mask DialogControl PLCBlockTitle Prompt: Core Variable Write
  wires:
  In1/1 -> __CoreVarWrite/1(u)

== system blending_tank_auto/PLC Controller/__Logic/Task/Program/__Logic/CTU/RungInOverride/ForceRungInFalseRead/__CoreLabelRead ==
  DataRead : DataStoreRead  DataStoreName=x_PLCLabel__s4_3653__Force_RungIn_False
  Out1 : Outport  VectorParamsAs1DForOutWhenUnconnected=off
  wires:
  DataRead/1 -> Out1/1

== system blending_tank_auto/PLC Controller/__Logic/Task/Program/__Logic/EQU/RungInOverride/ForceRungInFalseRead/__CoreLabelRead ==
  DataRead : DataStoreRead  DataStoreName=x_PLCLabel__s4_3653__Force_RungIn_False
  Out1 : Outport  VectorParamsAs1DForOutWhenUnconnected=off
  wires:
  DataRead/1 -> Out1/1

== system blending_tank_auto/PLC Controller/__Logic/Task/Program/__Logic/LEQ_1/RungInOverride/ForceRungInFalseRead/__CoreLabelRead ==
  DataRead : DataStoreRead  DataStoreName=x_PLCLabel__s4_3653__Force_RungIn_False
  Out1 : Outport  VectorParamsAs1DForOutWhenUnconnected=off
  wires:
  DataRead/1 -> Out1/1

== system blending_tank_auto/PLC Controller/__Logic/Task/Program/__Logic/LEQ_2/RungInOverride/ForceRungInFalseRead/__CoreLabelRead ==
  DataRead : DataStoreRead  DataStoreName=x_PLCLabel__s4_3653__Force_RungIn_False
  Out1 : Outport  VectorParamsAs1DForOutWhenUnconnected=off
  wires:
  DataRead/1 -> Out1/1

== system blending_tank_auto/PLC Controller/__Logic/Task/Program/__Logic/LEQ_3/RungInOverride/ForceRungInFalseRead/__CoreLabelRead ==
  DataRead : DataStoreRead  DataStoreName=x_PLCLabel__s4_3653__Force_RungIn_False
  Out1 : Outport  VectorParamsAs1DForOutWhenUnconnected=off
  wires:
  DataRead/1 -> Out1/1

== system blending_tank_auto/PLC Controller/__Logic/Task/Program/__Logic/LEQ_4/RungInOverride/ForceRungInFalseRead/__CoreLabelRead ==
  DataRead : DataStoreRead  DataStoreName=x_PLCLabel__s4_3653__Force_RungIn_False
  Out1 : Outport  VectorParamsAs1DForOutWhenUnconnected=off
  wires:
  DataRead/1 -> Out1/1

== system blending_tank_auto/PLC Controller/__Logic/Task/Program/__Logic/OTE/Instruction_Enable/Initialize Function/__CoreVarWrite ==
  u : Inport
  DataWrite : DataStoreWrite  DataStoreName=xxx_PLC_VAR_Initialise
  wires:
  u/1 -> DataWrite/1

== system blending_tank_auto/PLC Controller/__Logic/Task/Program/__Logic/OTE/Instruction_Enable/Rung-condition is false/__CoreVarWrite ==
  u : Inport
  DataWrite : DataStoreWrite  DataStoreName=xxx_PLC_VAR_Initialise
  wires:
  u/1 -> DataWrite/1

== system blending_tank_auto/PLC Controller/__Logic/Task/Program/__Logic/OTE/Instruction_Enable/Rung-condition-in is true/__CoreVarWrite ==
  u : Inport
  DataWrite : DataStoreWrite  DataStoreName=xxx_PLC_VAR_Initialise
  wires:
  u/1 -> DataWrite/1

== system blending_tank_auto/PLC Controller/__Logic/Task/Program/__Logic/OTE/RungInOverride/ForceRungInFalseRead/__CoreLabelRead ==
  DataRead : DataStoreRead  DataStoreName=x_PLCLabel__s4_3653__Force_RungIn_False
  Out1 : Outport  VectorParamsAs1DForOutWhenUnconnected=off
  wires:
  DataRead/1 -> Out1/1

== system blending_tank_auto/PLC Controller/__Logic/Task/Program/__Logic/OTE1/Instruction_Enable/Initialize Function/__CoreVarWrite ==
  u : Inport
  DataWrite : DataStoreWrite  DataStoreName=xxx_PLC_VAR_IV1_Signal
  wires:
  u/1 -> DataWrite/1

== system blending_tank_auto/PLC Controller/__Logic/Task/Program/__Logic/OTE1/Instruction_Enable/Rung-condition is false/__CoreVarWrite ==
  u : Inport
  DataWrite : DataStoreWrite  DataStoreName=xxx_PLC_VAR_IV1_Signal
  wires:
  u/1 -> DataWrite/1

== system blending_tank_auto/PLC Controller/__Logic/Task/Program/__Logic/OTE1/Instruction_Enable/Rung-condition-in is true/__CoreVarWrite ==
  u : Inport
  DataWrite : DataStoreWrite  DataStoreName=xxx_PLC_VAR_IV1_Signal
  wires:
  u/1 -> DataWrite/1

== system blending_tank_auto/PLC Controller/__Logic/Task/Program/__Logic/OTE1/RungInOverride/ForceRungInFalseRead/__CoreLabelRead ==
  DataRead : DataStoreRead  DataStoreName=x_PLCLabel__s4_3653__Force_RungIn_False
  Out1 : Outport  VectorParamsAs1DForOutWhenUnconnected=off
  wires:
  DataRead/1 -> Out1/1

== system blending_tank_auto/PLC Controller/__Logic/Task/Program/__Logic/OTE2/Instruction_Enable/Initialize Function/__CoreVarWrite ==
  u : Inport
  DataWrite : DataStoreWrite  DataStoreName=xxx_PLC_VAR_IV2_Signal
  wires:
  u/1 -> DataWrite/1

== system blending_tank_auto/PLC Controller/__Logic/Task/Program/__Logic/OTE2/Instruction_Enable/Rung-condition is false/__CoreVarWrite ==
  u : Inport
  DataWrite : DataStoreWrite  DataStoreName=xxx_PLC_VAR_IV2_Signal
  wires:
  u/1 -> DataWrite/1

== system blending_tank_auto/PLC Controller/__Logic/Task/Program/__Logic/OTE2/Instruction_Enable/Rung-condition-in is true/__CoreVarWrite ==
  u : Inport
  DataWrite : DataStoreWrite  DataStoreName=xxx_PLC_VAR_IV2_Signal
  wires:
  u/1 -> DataWrite/1

== system blending_tank_auto/PLC Controller/__Logic/Task/Program/__Logic/OTE2/RungInOverride/ForceRungInFalseRead/__CoreLabelRead ==
  DataRead : DataStoreRead  DataStoreName=x_PLCLabel__s4_3653__Force_RungIn_False
  Out1 : Outport  VectorParamsAs1DForOutWhenUnconnected=off
  wires:
  DataRead/1 -> Out1/1

== system blending_tank_auto/PLC Controller/__Logic/Task/Program/__Logic/OTE3/Instruction_Enable/Initialize Function/__CoreVarWrite ==
  u : Inport
  DataWrite : DataStoreWrite  DataStoreName=xxx_PLC_VAR_IV3_Signal
  wires:
  u/1 -> DataWrite/1

== system blending_tank_auto/PLC Controller/__Logic/Task/Program/__Logic/OTE3/Instruction_Enable/Rung-condition is false/__CoreVarWrite ==
  u : Inport
  DataWrite : DataStoreWrite  DataStoreName=xxx_PLC_VAR_IV3_Signal
  wires:
  u/1 -> DataWrite/1

== system blending_tank_auto/PLC Controller/__Logic/Task/Program/__Logic/OTE3/Instruction_Enable/Rung-condition-in is true/__CoreVarWrite ==
  u : Inport
  DataWrite : DataStoreWrite  DataStoreName=xxx_PLC_VAR_IV3_Signal
  wires:
  u/1 -> DataWrite/1

== system blending_tank_auto/PLC Controller/__Logic/Task/Program/__Logic/OTE3/RungInOverride/ForceRungInFalseRead/__CoreLabelRead ==
  DataRead : DataStoreRead  DataStoreName=x_PLCLabel__s4_3653__Force_RungIn_False
  Out1 : Outport  VectorParamsAs1DForOutWhenUnconnected=off
  wires:
  DataRead/1 -> Out1/1

== system blending_tank_auto/PLC Controller/__Logic/Task/Program/__Logic/OTE4/Instruction_Enable/Initialize Function/__CoreVarWrite ==
  u : Inport
  DataWrite : DataStoreWrite  DataStoreName=xxx_PLC_VAR_IV4_Signal
  wires:
  u/1 -> DataWrite/1

== system blending_tank_auto/PLC Controller/__Logic/Task/Program/__Logic/OTE4/Instruction_Enable/Rung-condition is false/__CoreVarWrite ==
  u : Inport
  DataWrite : DataStoreWrite  DataStoreName=xxx_PLC_VAR_IV4_Signal
  wires:
  u/1 -> DataWrite/1

== system blending_tank_auto/PLC Controller/__Logic/Task/Program/__Logic/OTE4/Instruction_Enable/Rung-condition-in is true/__CoreVarWrite ==
  u : Inport
  DataWrite : DataStoreWrite  DataStoreName=xxx_PLC_VAR_IV4_Signal
  wires:
  u/1 -> DataWrite/1

== system blending_tank_auto/PLC Controller/__Logic/Task/Program/__Logic/OTE4/RungInOverride/ForceRungInFalseRead/__CoreLabelRead ==
  DataRead : DataStoreRead  DataStoreName=x_PLCLabel__s4_3653__Force_RungIn_False
  Out1 : Outport  VectorParamsAs1DForOutWhenUnconnected=off
  wires:
  DataRead/1 -> Out1/1

== system blending_tank_auto/PLC Controller/__Logic/Task/Program/__Logic/OTE5/Instruction_Enable/Initialize Function/__CoreVarWrite ==
  u : Inport
  DataWrite : DataStoreWrite  DataStoreName=xxx_PLC_VAR_OV_Signal
  wires:
  u/1 -> DataWrite/1

== system blending_tank_auto/PLC Controller/__Logic/Task/Program/__Logic/OTE5/Instruction_Enable/Rung-condition is false/__CoreVarWrite ==
  u : Inport
  DataWrite : DataStoreWrite  DataStoreName=xxx_PLC_VAR_OV_Signal
  wires:
  u/1 -> DataWrite/1

== system blending_tank_auto/PLC Controller/__Logic/Task/Program/__Logic/OTE5/Instruction_Enable/Rung-condition-in is true/__CoreVarWrite ==
  u : Inport
  DataWrite : DataStoreWrite  DataStoreName=xxx_PLC_VAR_OV_Signal
  wires:
  u/1 -> DataWrite/1

== system blending_tank_auto/PLC Controller/__Logic/Task/Program/__Logic/OTE5/RungInOverride/ForceRungInFalseRead/__CoreLabelRead ==
  DataRead : DataStoreRead  DataStoreName=x_PLCLabel__s4_3653__Force_RungIn_False
  Out1 : Outport  VectorParamsAs1DForOutWhenUnconnected=off
  wires:
  DataRead/1 -> Out1/1

== system blending_tank_auto/PLC Controller/__Logic/Task/Program/__Logic/OTE6/Instruction_Enable/Initialize Function/__CoreVarWrite ==
  u : Inport
  DataWrite : DataStoreWrite  DataStoreName=xxx_PLC_VAR_Stirrer_Signal
  wires:
  u/1 -> DataWrite/1

== system blending_tank_auto/PLC Controller/__Logic/Task/Program/__Logic/OTE6/Instruction_Enable/Rung-condition is false/__CoreVarWrite ==
  u : Inport
  DataWrite : DataStoreWrite  DataStoreName=xxx_PLC_VAR_Stirrer_Signal
  wires:
  u/1 -> DataWrite/1

== system blending_tank_auto/PLC Controller/__Logic/Task/Program/__Logic/OTE6/Instruction_Enable/Rung-condition-in is true/__CoreVarWrite ==
  u : Inport
  DataWrite : DataStoreWrite  DataStoreName=xxx_PLC_VAR_Stirrer_Signal
  wires:
  u/1 -> DataWrite/1
